simulink model "QPSK"  (R2017b)
settings: Solver=VariableStepAuto  StartTime=0.0  StopTime=10.0  RelTol=1e-3
libraries: dsparch4 x2, commrandsrc3 x2
settings Model: Creator=ayadd  LastModifiedBy=ayadd

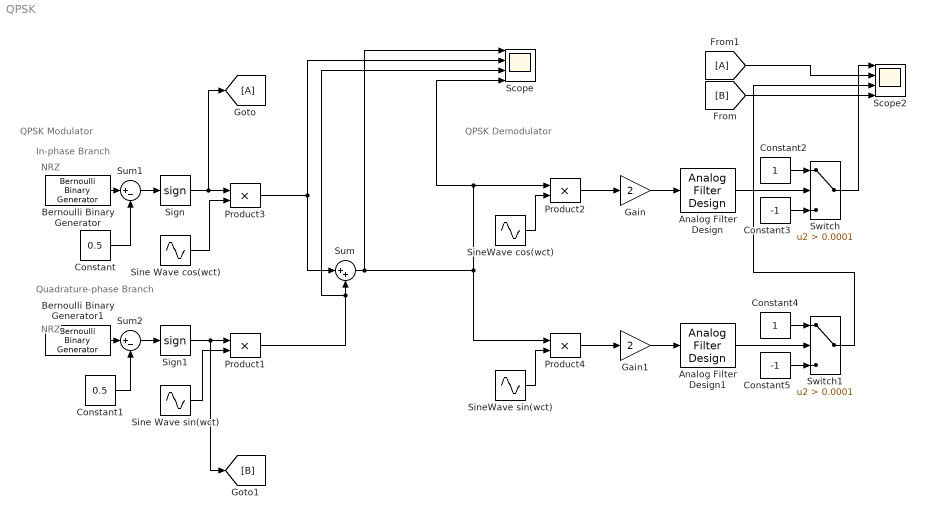
== system QPSK ==
  note: QPSK Demodulator
  note: QPSK Modulator
  note: In-phase Branch
  note: NRZ
  note: NRZ
  note: Quadrature-phase Branch
  Analog Filter Design : dsparch4/Analog Filter Design  method=Butterworth  filttype=Lowpass  N=8  Wlo=4*2*pi  Whi=80  Rp=2  Rs=40
  Analog Filter Design1 : dsparch4/Analog Filter Design  method=Butterworth  filttype=Lowpass  N=8  Wlo=4*2*pi  Whi=80  Rp=2  Rs=40
  Bernoulli Binary Generator : commrandsrc3/Bernoulli Binary Generator  ProbabilityOfZero=0.5  SeedSource=Auto  Seed=0  SampleTime=1  SamplesPerFrame=1  OutputDataType=double  SimulateUsing=Interpreted execution
  Bernoulli Binary Generator1 : commrandsrc3/Bernoulli Binary Generator  ProbabilityOfZero=0.5  SeedSource=Auto  Seed=0  SampleTime=1  SamplesPerFrame=1  OutputDataType=double  SimulateUsing=Interpreted execution
  Constant : Constant  Value=0.5
  Constant1 : Constant  Value=0.5
  Constant2 : Constant
  Constant3 : Constant  Value=-1
  Constant4 : Constant
  Constant5 : Constant  Value=-1
  Gain : Gain  Gain=2
  Gain1 : Gain  Gain=2
  Product{1..4} (4 alike) : Product  SaturateOnIntegerOverflow=on  InputSameDT=on  OutDataTypeStr=Inherit: Same as first input
  Scope : Scope  NumInputPorts=4
  Scope2 : Scope  NumInputPorts=4
  Sign : Signum
  Sign1 : Signum
  Sine Wave cos(‏wct) : Sin  Frequency=4*2*pi  Phase=pi/2  SampleTime=0.001
  Sine Wave sin(wct) : Sin  Amplitude=-1  Frequency=4*2*pi  SampleTime=0.001
  SineWave cos(‏wct) : Sin  Frequency=4*2*pi  Phase=pi/2  SampleTime=0.001
  SineWave sin(wct) : Sin  Amplitude=-1  Frequency=4*2*pi  SampleTime=0.001
  Sum : Sum  Inputs=|++
  Sum1 : Sum  Inputs=|+-
  Sum2 : Sum  Inputs=|+-
  Switch : Switch  Criteria=u2 > Threshold  Threshold=0.0001  RndMeth=Round  SaturateOnIntegerOverflow=on  InputSameDT=on
  Switch1 : Switch  Criteria=u2 > Threshold  Threshold=0.0001  RndMeth=Round  SaturateOnIntegerOverflow=on  InputSameDT=on
  wires:
  Sine Wave cos(‏wct)/1 -> Product3/2
  Sign/1 -> [A], Product3/1
  Sign1/1 -> Product1/1, [B]
  Sine Wave sin(wct)/1 -> Product1/2
  Product3/1 -> Scope/2, Sum/1
  Sum1/1 -> Sign/1
  Constant/1 -> Sum1/2
  Sum2/1 -> Sign1/1
  Bernoulli Binary Generator1/1 -> Sum2/1
  Constant1/1 -> Sum2/2
  Product1/1 -> Scope/3, Sum/2
  SineWave cos(‏wct)/1 -> Product2/2
  Product2/1 -> Gain/1
  SineWave sin(wct)/1 -> Product4/2
  Constant2/1 -> Switch/1
  Constant3/1 -> Switch/3
  Analog Filter Design/1 -> Switch/2
  Gain/1 -> Analog Filter Design/1
  Switch/1 -> Scope2/1
  Product4/1 -> Gain1/1
  Constant5/1 -> Switch1/3
  Analog Filter Design1/1 -> Switch1/2
  Constant4/1 -> Switch1/1
  Gain1/1 -> Analog Filter Design1/1
  [A] -> Scope2/2
  Switch1/1 -> Scope2/3
  [B] -> Scope2/4
  Sum/1 -> Product4/1, Scope/4, Product2/1, Scope/1
  Bernoulli Binary Generator/1 -> Sum1/1
